simulink model "control_comparison"  (R2023b)
settings: Solver=VariableStepAuto  StartTime=0.0  StopTime=30.0  RelTol=1e-3
values from neighbouring files (symbols this model uses):
  A = double(A)    [Rotational_inverted_pendulum.m]
  A_uns = double(A_uns)    [Rotational_inverted_pendulum.m]
  B = double(B)    [Rotational_inverted_pendulum.m]
  B_uns = double(B_uns)    [Rotational_inverted_pendulum.m]
  den_phi = cell2mat(G_t2p_uns.Denominator)    [Rotational_inverted_pendulum.m]
  den_theta = cell2mat(G_ol_uns.Denominator(1,1))    [Rotational_inverted_pendulum.m]
  K_pp = place(A,B,P)    [Rotational_inverted_pendulum.m]
  K_pp_uns = place(A_uns,B_uns,P_uns)    [Rotational_inverted_pendulum.m]
  Kd_phi = 60    [Rotational_inverted_pendulum.m]
  Kd_theta = 2    [Rotational_inverted_pendulum.m]
  Ki_phi = 50    [Rotational_inverted_pendulum.m]
  Ki_theta = 0    [Rotational_inverted_pendulum.m]
  Kp_phi = 90    [Rotational_inverted_pendulum.m]
  Kp_theta = 5    [Rotational_inverted_pendulum.m]
  num_phi = cell2mat(G_t2p_uns.Numerator)    [Rotational_inverted_pendulum.m]
  num_theta = cell2mat(G_ol_uns.Numerator(1,1))    [Rotational_inverted_pendulum.m]
  Va_bar = 0    [Rotational_inverted_pendulum.m]
  x1_bar = double(sol.x1)    [Rotational_inverted_pendulum.m]
  x1_bar_uns = x1_bar    [Rotational_inverted_pendulum.m]
  x3_bar = 0    [Rotational_inverted_pendulum.m]
  x3_bar_uns = pi    (= 3.14159265359)    [Rotational_inverted_pendulum.m]
undefined symbols (not defined in the file or in its folder): K_lq, K_lq_uns
libraries: simulink_extras x14, slpidlib x2, simulink x1
settings Model: Creator=Mark  LastModifiedBy=Mark

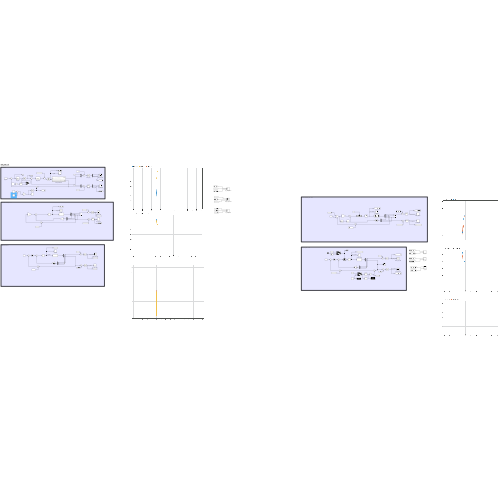
[thumbnail: Simulink's stored preview of the top-level diagram]
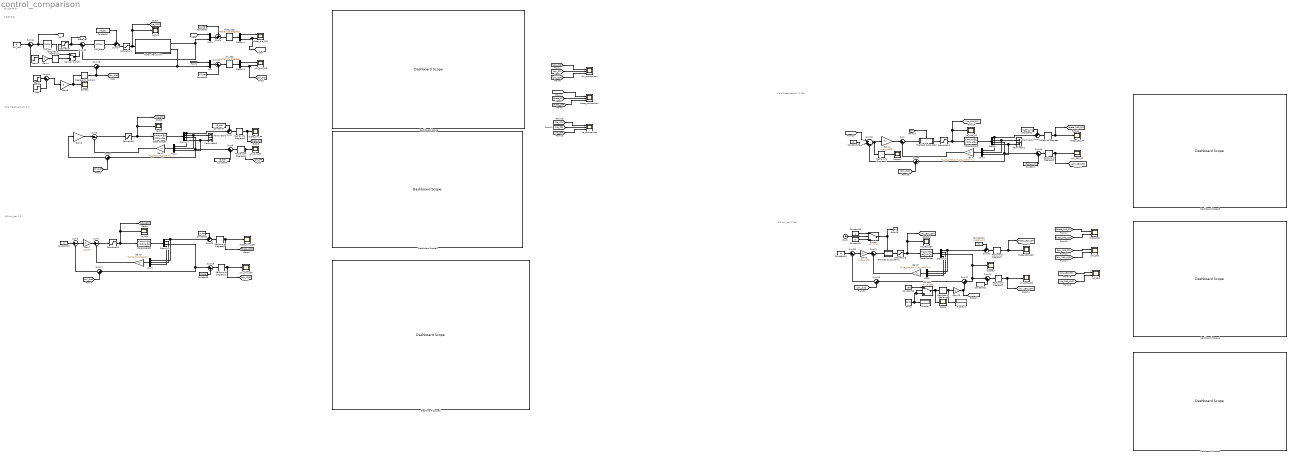
== system control_comparison ==
  note: phi_bar = 0°
  note: 2-DOF PID
  note: Pole Placement phi = 0
  note: LQR phi_bar = 0
  note: Pole Placement phi = 180
  note: LQR phi_bar = 180
  Clock : Clock
  Constant : Constant  Value=x3_bar_uns
  Constant1 : Constant  Value=x1_bar
  Constant10 : Constant  Value=0
  Constant11 : Constant  Value=x3_bar_uns
  Constant12 : Constant  Value=x1_bar_uns
  Constant13 : Constant
  Constant14 : Constant  Value=0
  Constant15 : Constant  Value=pi
  Constant16 : Constant  Value=180
  Constant17 : Constant  Value=pi
  Constant2 : Constant  Value=x1_bar_uns
  Constant3 : Constant  Value=x3_bar
  Constant4 : Constant  Value=x1_bar
  Constant6 : Constant  Value=x3_bar
  Constant7 : Constant  Value=Va_bar
  Constant8 : Constant  Value=x3_bar
  Constant9 : Constant  Value=x1_bar
  Dashboard Scope{,1..5} (6 alike) : DashboardScope
  Degrees to Radians : simulink_extras/Transformations/Degrees to Radians
  Degrees to Radians1 : simulink_extras/Transformations/Degrees to Radians
  Degrees to Radians4 : simulink_extras/Transformations/Degrees to Radians
  Demux{,1..2,5} (4 alike) : Demux
  Demux3 : Demux  Outputs=2
  Demux4 : Demux  Outputs=2
  Display : Display
  Display1 : Display
  Enabled Subsystem : Subsystem  TreatAsAtomicUnit=on
  Enabled Subsystem1 : Subsystem  TreatAsAtomicUnit=on
  From : From
  Gain : Gain  Gain=[K_pp_uns(1:2) K_pp_uns(4)]  Multiplication=Matrix(K*u) (u vector)
  Gain1 : Gain  Gain=K_pp_uns(3)
  Gain10 : Gain
  Gain2 : Gain  Gain=[K_pp(1:2) K_pp(4)]  Multiplication=Matrix(K*u) (u vector)
  Gain3 : Gain  Gain=K_pp(3)
  Gain4 : Gain
  Gain5 : Gain  Gain=[K_lq(1:2) K_lq(4)]  Multiplication=Matrix(K*u) (u vector)
  Gain6 : Gain  Gain=5
  Gain7 : Gain  Gain=K_lq(3)
  Gain8 : Gain  Gain=[K_lq_uns(1:2) K_lq_uns(4)]  Multiplication=Matrix(K*u) (u vector)
  Gain9 : Gain  Gain=K_lq_uns(3)
  Manual Switch1 : ManualSwitch
  Mux : Mux  Inputs=2
  Mux1 : Mux  Inputs=2
  Mux{2..5} (4 alike) : Mux  Inputs=3
  PID_phi : slpidlib/PID Controller  Controller=PID  Form=Parallel  TimeDomain=Continuous-time  UseExternalTs=off  SampleTime=-1  IntegratorMethod=Forward Euler  FilterMethod=Forward Euler  ControllerParametersSource=internal  P=Kp_phi  I=Ki_phi  UseKiTs=off  D=Kd_phi  N=100  UseFilter=on  TunerSelectOption=Transfer Function Based (PID Tuner App)  InitialConditionSource=internal  InitialConditionForIntegrator=0  InitialConditionForFilter=0  DifferentiatorICPrevScaledInput=0  ExternalReset=none  TrackingMode=off  Kt=1  LimitOutput=off  SatLimitsSource=internal  UpperSaturationLimit=90  LowerSaturationLimit=-90  LinearizeAsGain=on  AntiWindupMode=none  Kb=1  LimitIntegrator=off  UpperIntegratorSaturationLimit=inf  LowerIntegratorSaturationLimit=-inf  POutMin=[]  POutMax=[]  IOutMin=[]  IOutMax=[]  DOutMin=[]  DOutMax=[]  NOutMin=[]  NOutMax=[]  SumOutMin=[]  SumOutMax=[]  SaturationOutMin=[]  SaturationOutMax=[]  PParamMin=[]  PParamMax=[]  IParamMin=[]  IParamMax=[]  DParamMin=[]  DParamMax=[]  NParamMin=[]  NParamMax=[]  KbParamMin=[]  KbParamMax=[]  KtParamMin=[]  KtParamMax=[]  KbOutMin=[]  KbOutMax=[]  KtOutMin=[]  KtOutMax=[]  IntegratorOutMin=[]  IntegratorOutMax=[]  FilterOutMin=[]  FilterOutMax=[]  SumI1OutMin=[]  SumI1OutMax=[]  SumI2OutMin=[]  SumI2OutMax=[]  SumI3OutMin=[]  SumI3OutMax=[]  SumI4OutMin=[]  SumI4OutMax=[]  SumDOutMin=[]  SumDOutMax=[]  DifferentiatorOutMin=[]  DifferentiatorOutMax=[]  FilterDiffOutCoefMin=[]  FilterDiffOutCoefMax=[]  ReciprocalOutMin=[]  ReciprocalOutMax=[]  SumDenOutMin=[]  SumDenOutMax=[]  SumNumOutMin=[]  SumNumOutMax=[]  DivideOutMin=[]  DivideOutMax=[]  UdiffTsProdOutMin=[]  UdiffTsProdOutMax=[]  NTsProdOutMin=[]  NTsProdOutMax=[]  UintegralTsProdOutMin=[]  UintegralTsProdOutMax=[]  UngainTsProdOutMin=[]  UngainTsProdOutMax=[]  ClampingZeroOutDataTypeStr=Inherit: Inherit via back propagation  ClampingZeroOutMin=[]  ClampingZeroOutMax=[]  FilterDenConstantOutDataTypeStr=Inherit: Inherit via back propagation  FilterDenConstantOutMin=[]  FilterDenConstantOutMax=[]  PCopyOutDataTypeStr=Inherit: Inherit via back propagation  PCopyOutMin=[]  PCopyOutMax=[]  NCopyOutDataTypeStr=Inherit: Inherit via back propagation  NCopyOutMin=[]  NCopyOutMax=[]  IntegratorContinuousStateAttributes=''  IntegratorStateMustResolveToSignalObject=off  IntegratorRTWStateStorageClass=Auto  FilterContinuousStateAttributes=''  FilterStateMustResolveToSignalObject=off  FilterRTWStateStorageClass=Auto  ParallelPVariant=InternalParameters  IdealPVariant=Disabled  IVariant=InternalParameters  DVariant=InternalParameters  IntegratorVariant=Continuous  SatVariant=Disabled  AWVariant=Passthrough  PCopyVariant=Disabled  TRVariant=Disabled  FdbkBlocksVariant=Forward  IdealPFdbkVariant=Disabled  SatFdbkVariant=Disabled  DerivativeFilterVariant=ContFilter  NVariant=InternalParameters  NCopyVariant=Disabled  FilterICVariant=InternalICsFilter  IntegratorICVariant=InternalICs  ExternalResetVariant=Disabled  TRSumVariant=Passthrough  SumFdbkVariant=Disabled  SumVariant=Sum_PID  TsampFilterVariant=InternalTs  TsampNgainVariant=Passthrough  TsampIntegralVariant=Disabled_SignalSpec  ExternalSaturationOutDataTypeStr=Inherit: Same as second input
  PID_theta : slpidlib/PID Controller  Controller=PID  Form=Parallel  TimeDomain=Continuous-time  UseExternalTs=off  SampleTime=-1  IntegratorMethod=Forward Euler  FilterMethod=Forward Euler  ControllerParametersSource=internal  P=Kp_theta  I=Ki_theta  UseKiTs=off  D=Kd_theta  N=100  UseFilter=on  TunerSelectOption=Frequency Response Based  InitialConditionSource=internal  InitialConditionForIntegrator=0  InitialConditionForFilter=0  DifferentiatorICPrevScaledInput=0  ExternalReset=none  TrackingMode=off  Kt=1  LimitOutput=off  SatLimitsSource=internal  UpperSaturationLimit=10  LowerSaturationLimit=-10  LinearizeAsGain=on  AntiWindupMode=back-calculation  Kb=Ki_theta/Kp_theta  LimitIntegrator=off  UpperIntegratorSaturationLimit=inf  LowerIntegratorSaturationLimit=-inf  POutMin=[]  POutMax=[]  IOutMin=[]  IOutMax=[]  DOutMin=[]  DOutMax=[]  NOutMin=[]  NOutMax=[]  SumOutMin=[]  SumOutMax=[]  SaturationOutMin=[]  SaturationOutMax=[]  PParamMin=[]  PParamMax=[]  IParamMin=[]  IParamMax=[]  DParamMin=[]  DParamMax=[]  NParamMin=[]  NParamMax=[]  KbParamMin=[]  KbParamMax=[]  KtParamMin=[]  KtParamMax=[]  KbOutMin=[]  KbOutMax=[]  KtOutMin=[]  KtOutMax=[]  IntegratorOutMin=[]  IntegratorOutMax=[]  FilterOutMin=[]  FilterOutMax=[]  SumI1OutMin=[]  SumI1OutMax=[]  SumI2OutMin=[]  SumI2OutMax=[]  SumI3OutMin=[]  SumI3OutMax=[]  SumI4OutMin=[]  SumI4OutMax=[]  SumDOutMin=[]  SumDOutMax=[]  DifferentiatorOutMin=[]  DifferentiatorOutMax=[]  FilterDiffOutCoefMin=[]  FilterDiffOutCoefMax=[]  ReciprocalOutMin=[]  ReciprocalOutMax=[]  SumDenOutMin=[]  SumDenOutMax=[]  SumNumOutMin=[]  SumNumOutMax=[]  DivideOutMin=[]  DivideOutMax=[]  UdiffTsProdOutMin=[]  UdiffTsProdOutMax=[]  NTsProdOutMin=[]  NTsProdOutMax=[]  UintegralTsProdOutMin=[]  UintegralTsProdOutMax=[]  UngainTsProdOutMin=[]  UngainTsProdOutMax=[]  ClampingZeroOutDataTypeStr=Inherit: Inherit via back propagation  ClampingZeroOutMin=[]  ClampingZeroOutMax=[]  FilterDenConstantOutDataTypeStr=Inherit: Inherit via back propagation  FilterDenConstantOutMin=[]  FilterDenConstantOutMax=[]  PCopyOutDataTypeStr=Inherit: Inherit via back propagation  PCopyOutMin=[]  PCopyOutMax=[]  NCopyOutDataTypeStr=Inherit: Inherit via back propagation  NCopyOutMin=[]  NCopyOutMax=[]  IntegratorContinuousStateAttributes=''  IntegratorStateMustResolveToSignalObject=off  IntegratorRTWStateStorageClass=Auto  FilterContinuousStateAttributes=''  FilterStateMustResolveToSignalObject=off  FilterRTWStateStorageClass=Auto  ParallelPVariant=InternalParameters  IdealPVariant=Disabled  IVariant=InternalParameters  DVariant=InternalParameters  IntegratorVariant=Continuous  SatVariant=Disabled  AWVariant=Passthrough  PCopyVariant=Disabled  TRVariant=Disabled  FdbkBlocksVariant=Forward  IdealPFdbkVariant=Disabled  SatFdbkVariant=Disabled  DerivativeFilterVariant=ContFilter  NVariant=InternalParameters  NCopyVariant=Disabled  FilterICVariant=InternalICsFilter  IntegratorICVariant=InternalICs  ExternalResetVariant=Disabled  TRSumVariant=Passthrough  SumFdbkVariant=Disabled  SumVariant=Sum_PID  TsampFilterVariant=InternalTs  TsampNgainVariant=Passthrough  TsampIntegralVariant=Disabled_SignalSpec  ExternalSaturationOutDataTypeStr=Inherit: Same as second input
  Radians to Degrees{,1..8} (9 alike) : simulink_extras/Transformations/Radians to Degrees
  Ramp : simulink/Sources/Ramp  slope=50  start=0  InitialOutput=0
  Rotary Pendulum : Subsystem
  Saturation : Saturate  UpperLimit=pi/2  LowerLimit=-pi/2
  Saturation{1..5} (5 alike) : Saturate  UpperLimit=10  LowerLimit=-10
  Scope{,1,3..4} (4 alike) : Scope
  State-Space1 : StateSpace  A=A  B=B  C=eye(4)  D=zeros(4,1)  InitialCondition=[0 0 0 0]
  State-Space2 : StateSpace  A=A  B=B  C=eye(4)  D=zeros(4,1)  InitialCondition=[0 0 0 0]
  State-Space3 : StateSpace  A=A_uns  B=B_uns  C=[1 0 0 0; 0 1 0 0; 0 0 1 0; 0 0 0 1]  D=[0 0 0 0]'  InitialCondition=[0 0 0 0]
  State-Space4 : StateSpace  A=A_uns  B=B_uns  C=eye(4)  D=zeros(4,1)  InitialCondition=[ 0 0 0 0]
  Step : Step  Time=10.05  SampleTime=0
  Step1 : Step  Time=10  SampleTime=0
  Step2 : Step  SampleTime=0
  Sum{,2,7,10..11,15,21,26} (8 alike) : Sum  Inputs=|+-
  Sum{1,4,9,14,16,22} (6 alike) : Sum  Inputs=++|
  Sum{5..6,8,12..13,17..19,23..24,27} (11 alike) : Sum  Inputs=|++
  Sum20 : Sum  Inputs=|-+-
  Sum3 : Sum  Inputs=|--
  Switch : Switch  Threshold=5  SaturateOnIntegerOverflow=off  InputSameDT=off
  Switch1 : Switch  Threshold=180  SaturateOnIntegerOverflow=off  InputSameDT=off
  Terminator{,1..3} (4 alike) : Terminator
  Va_180 : Scope  NumInputPorts=2
  Va_180_LQR : Scope
  Va_180_PP : Scope
  Va_LQR : Scope
  Va_PID : Scope
  Va_PP : Scope
  Va_comparison : Scope  NumInputPorts=3
  phi_180 : Scope  NumInputPorts=2
  phi_180_LQR : Scope
  phi_180_PP : Scope
  phi_comparison : Scope  NumInputPorts=3
  phi_deg : simulink_extras/Transformations/Radians to Degrees
  phi_ref1 : Constant  Value=0
  phi_sim_LQR : Scope
  phi_sim_PID : Scope  NumInputPorts=2
  phi_sim_PP : Scope
  theta_180 : Scope  NumInputPorts=2
  theta_180_LQR : Scope
  theta_180_PP : Scope
  theta_comparison : Scope  NumInputPorts=3
  theta_deg : simulink_extras/Transformations/Radians to Degrees
  theta_ref : Goto
  theta_sim_LQR : Scope
  theta_sim_PID : Scope  NumInputPorts=2
  theta_sim_PP : Scope
  wires:
  Degrees to Radians1/1 -> Manual Switch1/2
  Rotary Pendulum/1(theta) -> Mux1/2, Sum10/2
  Constant7/1 -> Sum14/1
  Saturation/1 -> theta_ref/1, Sum10/1
  PID_phi/1 -> Manual Switch1/1
  Step2/1 -> Gain4/1
  Sum15/1 -> Gain6/1
  Demux4/2 -> [theta_PID], theta_sim_PID/2  "theta_PID"
  Manual Switch1/1 -> Saturation/1
  Saturation1/1 -> [Va_PID], Va_PID/1, Rotary Pendulum/1(Va)  "Va_PID"
  Step1/1 -> Sum15/1
  Constant8/1 -> Sum12/2
  Mux1/1 -> Sum9/2
  Demux4/1 -> theta_sim_PID/1
  Sum11/1 -> [B], PID_phi/1
  theta_deg/1 -> Demux4/1
  Degrees to Radians/1 -> [phi_dist], Sum13/2
  Sum9/1 -> theta_deg/1
  Demux3/2 -> [phi_PID], phi_sim_PID/2  "phi_PID"
  Step/1 -> Sum15/2
  Mux/1 -> Sum12/1
  Rotary Pendulum/2(phi) -> Sum13/1, Mux/2
  From/1 -> Mux1/1
  Sum10/1 -> PID_theta/1
  phi_deg/1 -> Demux3/1
  Gain6/1 -> Scope1/1, Degrees to Radians/1
  Demux3/1 -> phi_sim_PID/1
  Sum12/1 -> phi_deg/1
  Constant9/1 -> Sum9/1
  phi_ref1/1 -> Sum11/1
  PID_theta/1 -> Sum14/2
  Gain4/1 -> Degrees to Radians1/1
  Sum13/1 -> Sum11/2
  Sum14/1 -> Saturation1/1
  [B] -> Mux/1
  Demux1/1 -> Mux2/1, Sum4/2
  Sum6/1 -> Radians to Degrees4/1
  Sum3/1 -> Saturation2/1
  Sum4/1 -> Radians to Degrees3/1
  Radians to Degrees3/1 -> [theta_PP], theta_sim_PP/1  "theta_PP"
  Gain3/1 -> Sum3/1
  Demux1/4 -> Mux2/3, Terminator3/1
  Sum5/1 -> Gain3/1
  Constant4/1 -> Sum4/1
  Gain2/1 -> Sum3/2
  Demux1/2 -> Mux2/2, Terminator2/1
  Radians to Degrees4/1 -> [phi_PP], phi_sim_PP/1  "phi_PP"
  Saturation2/1 -> State-Space1/1, Va_PP/1, [Va_PP]  "Va_PP"
  Constant3/1 -> Sum6/2
  Mux2/1 -> Gain2/1
  State-Space1/1 -> Demux1/1
  Demux1/3 -> Sum6/1, Sum5/1
  Radians to Degrees1/1 -> [phi_LQR], phi_sim_LQR/1  "phi_LQR"
  Constant6/1 -> Sum18/2
  Mux3/1 -> Gain5/1
  Sum17/1 -> Sum2/2
  Demux2/1 -> Sum16/2, Mux3/1
  Sum2/1 -> Gain7/1
  Demux2/2 -> Mux3/2
  Demux2/4 -> Mux3/3
  Constant1/1 -> Sum16/1
  Sum16/1 -> Radians to Degrees2/1
  Sum18/1 -> Radians to Degrees1/1
  Saturation3/1 -> State-Space2/1, [Va_LQR], Va_LQR/1  "Va_LQR"
  Gain5/1 -> Sum7/2
  State-Space2/1 -> Demux2/1
  Radians to Degrees2/1 -> theta_sim_LQR/1, [theta_LQR]  "theta_LQR"
  Gain7/1 -> Sum7/1
  Constant10/1 -> Sum2/1
  Sum7/1 -> Saturation3/1
  Demux2/3 -> Sum17/1, Sum18/1
  [phi_dist] -> Sum5/2
  [phi_dist] -> Sum17/2
  [phi_PID] -> phi_comparison/1
  [phi_PP] -> phi_comparison/2
  [phi_LQR] -> phi_comparison/3
  [theta_PID] -> theta_comparison/1
  [theta_PP] -> theta_comparison/2
  [theta_LQR] -> theta_comparison/3
  [Va_PID] -> Va_comparison/1
  [Va_PP] -> Va_comparison/2
  [Va_LQR] -> Va_comparison/3
  Demux/4 -> Mux4/3, Terminator1/1
  Sum/1 -> Enabled Subsystem/1(In1)
  Radians to Degrees6/1 -> Scope4/1
  Radians to Degrees/1 -> theta_180_PP/1, [theta_180_PP]  "theta_180_PP"
  Sum1/1 -> Radians to Degrees/1
  Sum20/1 -> Gain1/1, Radians to Degrees6/1
  Saturation4/1 -> State-Space3/1, Va_180_PP/1, [Va_180_PP]  "Va_180_PP"
  Demux/2 -> Mux4/2, Terminator/1
  Constant/1 -> Sum19/2
  Enabled Subsystem/1(Out1) -> Saturation4/1
  Radians to Degrees5/1 -> phi_180_PP/1, [phi_180_PP]  "phi_180_PP"
  Constant2/1 -> Sum1/1
  Mux4/1 -> Gain/1
  Gain/1 -> Sum/2
  Demux/1 -> Mux4/1, Sum1/2
  Constant17/1 -> Sum20/2
  Demux/3 -> Sum19/1, Sum8/1
  Sum8/1 -> Sum20/3
  Gain1/1 -> Sum/1
  State-Space3/1 -> Demux/1
  Sum19/1 -> Radians to Degrees5/1
  Radians to Degrees8/1 -> [phi_180_LQR], phi_180_LQR/1  "phi_180_LQR"
  Sum27/1 -> Sum23/1
  Demux5/1 -> Sum22/2, Mux5/1
  Demux5/2 -> Mux5/2
  Radians to Degrees7/1 -> [theta_180_LQR], theta_180_LQR/1  "theta_180_LQR"
  Demux5/4 -> Mux5/3
  Sum26/1 -> Gain9/1
  Clock/1 -> Switch/2
  Enabled Subsystem1/1(Out1) -> Saturation5/1
  Constant12/1 -> Sum22/1
  Constant16/1 -> Switch1/1
  Gain8/1 -> Sum21/2
  Constant13/1 -> Switch/1
  Ramp/1 -> Switch1/2, Switch1/3, Display/1
  Sum22/1 -> Radians to Degrees7/1
  Constant14/1 -> Switch/3
  Sum21/1 -> Enabled Subsystem1/1(In1)
  Mux5/1 -> Gain8/1
  Constant15/1 -> Sum26/1
  Sum24/1 -> Radians to Degrees8/1
  Demux5/3 -> Scope3/1, Sum27/1, Sum24/1
  Sum23/1 -> Sum26/2
  Gain9/1 -> Sum21/1
  State-Space4/1 -> Demux5/1
  Switch1/1 -> Scope/1, Degrees to Radians4/1
  Saturation5/1 -> State-Space4/1, Va_180_LQR/1, [Va_180_LQR]  "Va_180_LQR"
  Constant11/1 -> Sum24/2
  Gain10/1 -> [rising_phi], Sum27/2
  Switch/1 -> Enabled Subsystem1/Enable, [en]
  Degrees to Radians4/1 -> Display1/1, Gain10/1
  [phi_dist] -> Sum8/2
  [theta_180_PP] -> theta_180/1
  [theta_180_LQR] -> theta_180/2
  [phi_180_PP] -> phi_180/1
  [phi_180_LQR] -> phi_180/2
  [Va_180_PP] -> Va_180/1
  [Va_180_LQR] -> Va_180/2
  [rising_phi] -> Sum20/1
  [en] -> Enabled Subsystem/Enable
  [phi_dist] -> Sum23/2

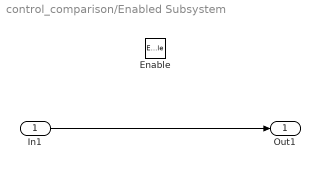
== system control_comparison/Enabled Subsystem ==
  In1 : Inport
  Enable : EnablePort
  Out1 : Outport
  wires:
  In1/1 -> Out1/1

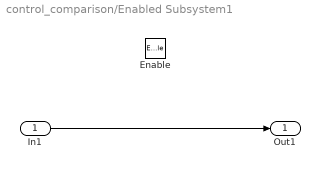
== system control_comparison/Enabled Subsystem1 ==
  In1 : Inport
  Enable : EnablePort
  Out1 : Outport
  wires:
  In1/1 -> Out1/1

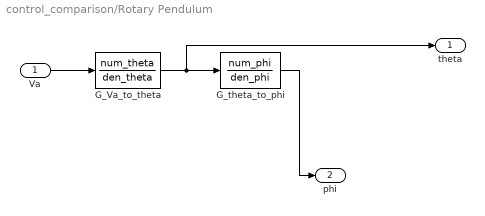
== system control_comparison/Rotary Pendulum ==
  Va : Inport
  G_Va_to_theta : TransferFcn  Numerator=num_theta  Denominator=den_theta
  G_theta_to_phi : TransferFcn  Numerator=num_phi  Denominator=den_phi
  theta : Outport
  phi : Outport  Port=2
  wires:
  G_theta_to_phi/1 -> phi/1
  G_Va_to_theta/1 -> theta/1, G_theta_to_phi/1
  Va/1 -> G_Va_to_theta/1
